simulink subsystem "HIL_Receive_TCP_Data_2021a"  (R2021b)
settings: Solver=VariableStepAuto  StartTime=0.0  StopTime=10.0  RelTol=1e-3
model mask{mi_ip=0, mi_port=0, f=0}
  mask prompts: mi_ip "Server IP"; mi_port "Server PORT"; f "Sampling Frequency"
libraries: slrealtimeiplib x2, slrealtimeutilitieslib x1
settings Model: Creator=ramuj  LastModifiedBy=Hyperloop UPV
settings DebuggingCC: UnconnectedInputMsg=none  UnconnectedOutputMsg=none  UnconnectedLineMsg=none
settings ModelReferenceCC: EnableRefExpFcnMdlSchedulingChecks=off
settings RTWCC: DLArmComputeVersion=20.02.1

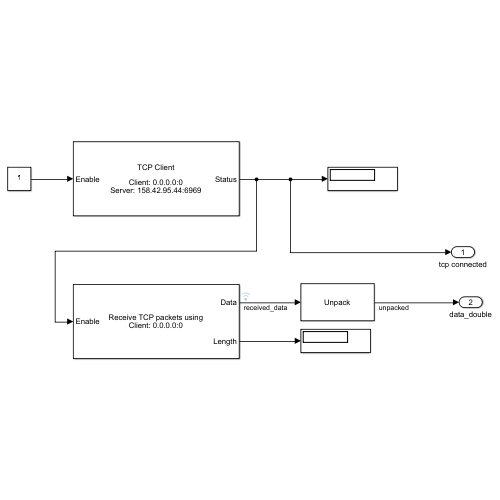
[thumbnail: Simulink's stored preview of the top-level diagram]
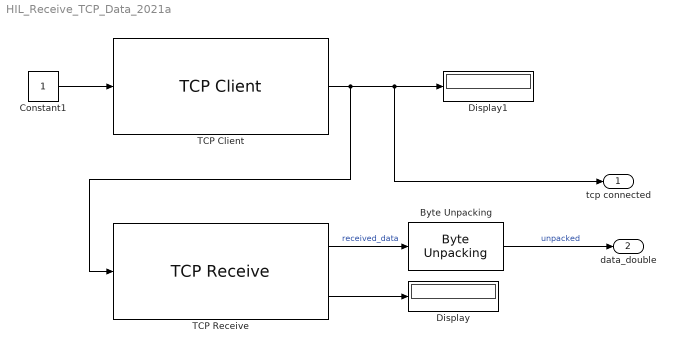
== system HIL_Receive_TCP_Data_2021a ==
  Byte Unpacking : slrealtimeutilitieslib/Byte Unpacking  MaskUnpackedDataTypes={'double'}  MaskUnpackedDataSizes={[1]}  MaskAlignment=1
      settings: SourceProductBaseCode=XP
  Constant1 : Constant
  Display : Display
  Display1 : Display
  TCP Client : slrealtimeiplib/TCP Client  Priority=-1  useHostTargetConn=off  remoteAddress='158.42.95.44'  remotePort=6969  clientAddress=0.0.0.0  clientPort=0
      settings: SourceProductBaseCode=XP
  TCP Receive : slrealtimeiplib/TCP Receive  socketAddPortVal=Client: 0.0.0.0:0  rcvWidth=8  sampleTime=1/f
      settings: SourceProductBaseCode=XP
  tcp connected : Outport
  data_double : Outport  Port=2  OutDataTypeStr=double
  wires:
  Constant1/1 -> TCP Client/1
  TCP Client/1 -> TCP Receive/1, Display1/1, tcp connected/1
  TCP Receive/2 -> Display/1
  TCP Receive/1 -> Byte Unpacking/1  "received_data"
  Byte Unpacking/1 -> data_double/1  "unpacked"
